simulink model "MDOF_WD"  (R2023a)
settings: Solver=VariableStepAuto  StartTime=0.0  StopTime=window  FixedStep=SimStep  RelTol=1e-3
values from neighbouring files (symbols this model uses):
  SimStep = 0.01    [Part1_01_Geneartion_Configuration.m]
undefined symbols (not defined in the file or in its folder): Aw, Bw, Cw, Dw, me
settings Model: Creator=cuishuaiwen  LastModifiedBy=cuishuaiwen
settings OptimizationCC: ReuseModelBlockBuffer=off

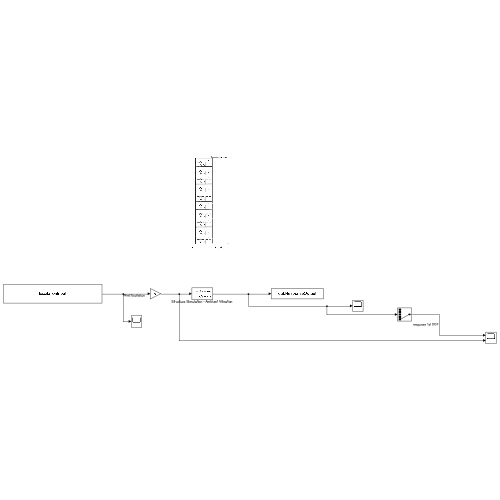
[thumbnail: Simulink's stored preview of the top-level diagram]
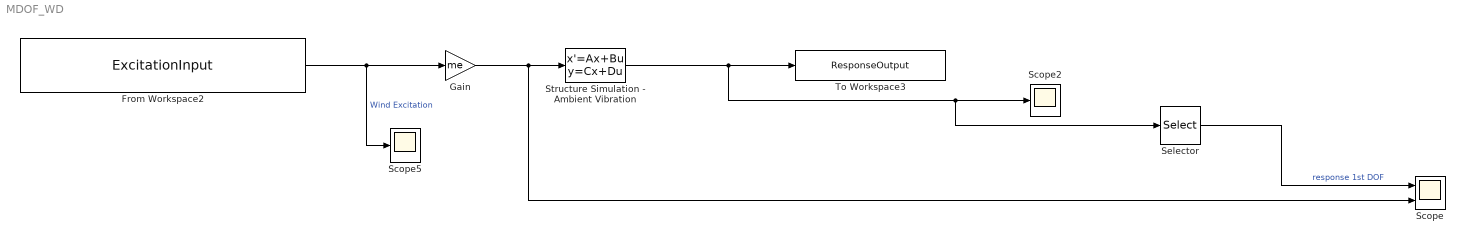
== system MDOF_WD ==
  From Workspace2 : FromWorkspace  VariableName=ExcitationInput  SampleTime=SimStep
  Gain : Gain  Gain=me
  Scope : Scope  NumInputPorts=2
  Scope2 : Scope
  Scope5 : Scope
  Selector : Selector  InputPortWidth=nDOF  IndexOptions=Index vector (dialog)  Indices=nDOF  OutputSizes=1
  Structure Simulation - Ambient Vibration : StateSpace  A=Aw  B=Bw  C=Cw  D=Dw  InitialCondition=0
  To Workspace3 : ToWorkspace  VariableName=ResponseOutput  SaveFormat=Structure With Time  SampleTime=SimStep
  wires:
  Structure Simulation - Ambient Vibration/1 -> Selector/1, Scope2/1, To Workspace3/1
  Selector/1 -> Scope/1  "response 1st DOF"
  From Workspace2/1 -> Gain/1, Scope5/1  "Wind Excitation"
  Gain/1 -> Scope/2, Structure Simulation - Ambient Vibration/1
